simulink model "project_simu"  (R2019a)
settings: Solver=VariableStepAuto  StartTime=0.0  StopTime=1  RelTol=1e-3
values from neighbouring files (symbols this model uses):
  banks = 1e6*banks_data    [project.m]
  f = Filters/mean(Filters)    [project.m]
  lines = lines_data    [project.m]
  loads = zeros(10,2)    [project.m]
  m = 2    [project.m]
libraries: powerlib x87, powerlib_meascontrol x1, sps_avr x1
(part 2 of 2)

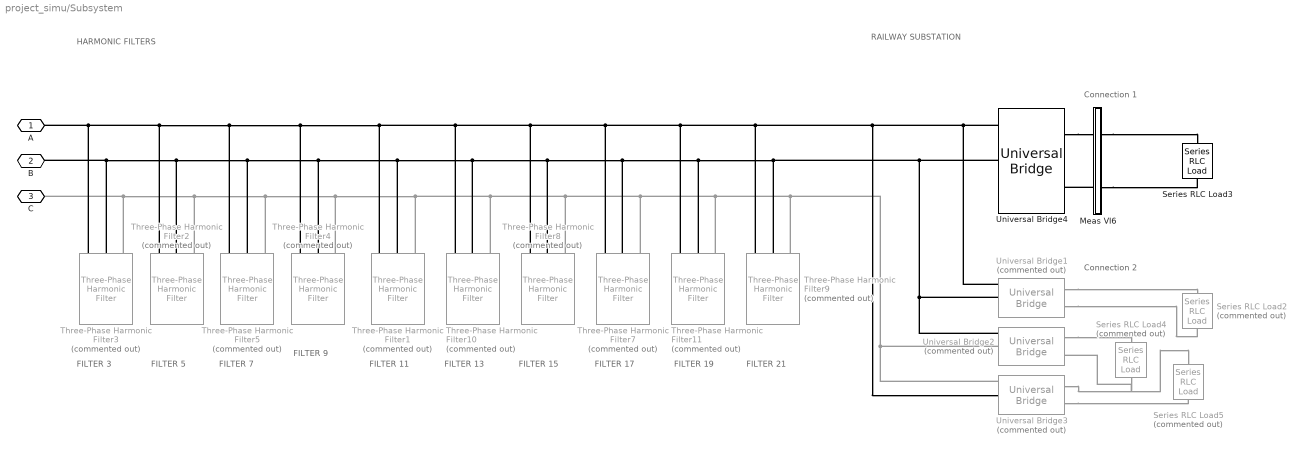
== system project_simu/Subsystem ==
  note: FILTER 5
  note: FILTER 11
  note: FILTER 3
  note: FILTER 9
  note: FILTER 7
  note: HARMONIC FILTERS
  note: RAILWAY SUBSTATION
  note: FILTER 17
  note: FILTER 15
  note: FILTER 21
  note: FILTER 13
  note: FILTER 19
  note: Connection 1
  note: Connection 2
  Meas VI6 : Subsystem
  Series RLC Load2 : powerlib/Elements/Series RLC Load  Commented=on  LConnTagsString=a  RConnTagsString=__new0  NominalVoltage=70e3*sqrt(2)  NominalFrequency=50  ActivePower=loads(10,1)/3  InductivePower=loads(10,2)/3  CapacitivePower=0  Setx0=off  InitialVoltage=0  SetiL0=off  InitialCurrent=0  Measurements=None  LoadType=constant Z
      settings: SourceProductName=Simscape Electrical
  Series RLC Load3 : powerlib/Elements/Series RLC Load  LConnTagsString=a  RConnTagsString=__new0  NominalVoltage=70e3*sqrt(2)  NominalFrequency=50  ActivePower=loads(10,1)  InductivePower=loads(10,2)  CapacitivePower=0  Setx0=off  InitialVoltage=0  SetiL0=off  InitialCurrent=0  Measurements=None  LoadType=constant Z
      settings: SourceProductName=Simscape Electrical
  Series RLC Load4 : powerlib/Elements/Series RLC Load  Commented=on  LConnTagsString=a  RConnTagsString=__new0  NominalVoltage=70e3*sqrt(2)  NominalFrequency=50  ActivePower=loads(10,1)/3  InductivePower=loads(10,2)/3  CapacitivePower=0  Setx0=off  InitialVoltage=0  SetiL0=off  InitialCurrent=0  Measurements=None  LoadType=constant Z
      settings: SourceProductName=Simscape Electrical
  Series RLC Load5 : powerlib/Elements/Series RLC Load  Commented=on  LConnTagsString=a  RConnTagsString=__new0  NominalVoltage=70e3*sqrt(2)  NominalFrequency=50  ActivePower=loads(10,1)/3  InductivePower=loads(10,2)/3  CapacitivePower=0  Setx0=off  InitialVoltage=0  SetiL0=off  InitialCurrent=0  Measurements=None  LoadType=constant Z
      settings: SourceProductName=Simscape Electrical
  Three-Phase Harmonic Filter1 : powerlib/Elements/Three-Phase Harmonic Filter  Commented=on  LConnTagsString=A|B|C  FilterType=Single-tuned  FilterConnection=Y (grounded)  ParNom=[70e3 50]  Qc=9e6*f(5)  Fr=[11*50]  Frd=[11*60 13*60]  Q=10  Measurements=None
      settings: AttributesFormatString=\n  SourceProductName=Simscape Electrical  SourceProductBaseCode=PS
  Three-Phase Harmonic Filter10 : powerlib/Elements/Three-Phase Harmonic Filter  Commented=on  LConnTagsString=A|B|C  FilterType=Single-tuned  FilterConnection=Y (grounded)  ParNom=[70e3 50]  Qc=9e6*f(6)  Fr=[13*50]  Frd=[11*60 13*60]  Q=10  Measurements=None
      settings: AttributesFormatString=\n  SourceProductName=Simscape Electrical  SourceProductBaseCode=PS
  Three-Phase Harmonic Filter11 : powerlib/Elements/Three-Phase Harmonic Filter  Commented=on  LConnTagsString=A|B|C  FilterType=Single-tuned  FilterConnection=Y (grounded)  ParNom=[70e3 50]  Qc=9e6*f(9)  Fr=[19*50]  Frd=[11*60 13*60]  Q=10  Measurements=None
      settings: AttributesFormatString=\n  SourceProductName=Simscape Electrical  SourceProductBaseCode=PS
  Three-Phase Harmonic Filter2 : powerlib/Elements/Three-Phase Harmonic Filter  Commented=on  LConnTagsString=A|B|C  FilterType=Single-tuned  FilterConnection=Y (grounded)  ParNom=[70e3 50]  Qc=9e6*f(2)  Fr=[5*50]  Frd=[266 323]  Q=10  Measurements=None
      settings: AttributesFormatString=\n  SourceProductName=Simscape Electrical  SourceProductBaseCode=PS
  Three-Phase Harmonic Filter3 : powerlib/Elements/Three-Phase Harmonic Filter  Commented=on  LConnTagsString=A|B|C  FilterType=Single-tuned  FilterConnection=Y (grounded)  ParNom=[70e3 50]  Qc=9e6*f(1)  Fr=[3*50]  Frd=[11*60 13*60]  Q=10  Measurements=None
      settings: AttributesFormatString=\n  SourceProductName=Simscape Electrical  SourceProductBaseCode=PS
  Three-Phase Harmonic Filter4 : powerlib/Elements/Three-Phase Harmonic Filter  Commented=on  LConnTagsString=A|B|C  FilterType=Single-tuned  FilterConnection=Y (grounded)  ParNom=[70e3 50]  Qc=9e6/9*f(4)  Fr=[9*50]  Frd=[11*60 13*60]  Q=10  Measurements=None
      settings: AttributesFormatString=\n  SourceProductName=Simscape Electrical  SourceProductBaseCode=PS
  Three-Phase Harmonic Filter5 : powerlib/Elements/Three-Phase Harmonic Filter  Commented=on  LConnTagsString=A|B|C  FilterType=Single-tuned  FilterConnection=Y (grounded)  ParNom=[70e3 50]  Qc=9e6/9*f(3)  Fr=[7*50]  Frd=[5*50 7*50]  Q=10  Measurements=None
      settings: AttributesFormatString=\n  SourceProductName=Simscape Electrical  SourceProductBaseCode=PS
  Three-Phase Harmonic Filter7 : powerlib/Elements/Three-Phase Harmonic Filter  Commented=on  LConnTagsString=A|B|C  FilterType=Single-tuned  FilterConnection=Y (grounded)  ParNom=[70e3 50]  Qc=9e6*f(8)  Fr=[17*50]  Frd=[11*60 13*60]  Q=10  Measurements=None
      settings: AttributesFormatString=\n  SourceProductName=Simscape Electrical  SourceProductBaseCode=PS
  Three-Phase Harmonic Filter8 : powerlib/Elements/Three-Phase Harmonic Filter  Commented=on  LConnTagsString=A|B|C  FilterType=Single-tuned  FilterConnection=Y (grounded)  ParNom=[70e3 50]  Qc=9e6*f(7)  Fr=[15*50]  Frd=[11*60 13*60]  Q=10  Measurements=None
      settings: AttributesFormatString=\n  SourceProductName=Simscape Electrical  SourceProductBaseCode=PS
  Three-Phase Harmonic Filter9 : powerlib/Elements/Three-Phase Harmonic Filter  Commented=on  LConnTagsString=A|B|C  FilterType=Single-tuned  FilterConnection=Y (grounded)  ParNom=[70e3 50]  Qc=9e6*f(10)  Fr=[21*50]  Frd=[11*60 13*60]  Q=10  Measurements=None
      settings: AttributesFormatString=\n  SourceProductName=Simscape Electrical  SourceProductBaseCode=PS
  Universal Bridge1 : powerlib/Power Electronics/Universal Bridge  Commented=on  Arms=3  SnubberResistance=1e5  SnubberCapacitance=inf  Device=Diodes  Ron=1e-3  Lon=0  ForwardVoltages="[  0  0  ]"  ForwardVoltage=0  GTOparameters=[ 10e-6 , 20e-6 ]  IGBTparameters=[ 1e-6 , 2e-6 ]  Measurements=None  Measurements_2=None  converterType=Rectifier
      settings: SourceProductName=Simscape Electrical
  Universal Bridge2 : powerlib/Power Electronics/Universal Bridge  Commented=on  Arms=3  SnubberResistance=1e5  SnubberCapacitance=inf  Device=Diodes  Ron=1e-3  Lon=0  ForwardVoltages="[  0  0  ]"  ForwardVoltage=0  GTOparameters=[ 10e-6 , 20e-6 ]  IGBTparameters=[ 1e-6 , 2e-6 ]  Measurements=None  Measurements_2=None  converterType=Rectifier
      settings: SourceProductName=Simscape Electrical
  Universal Bridge3 : powerlib/Power Electronics/Universal Bridge  Commented=on  Arms=3  SnubberResistance=1e5  SnubberCapacitance=inf  Device=Diodes  Ron=1e-3  Lon=0  ForwardVoltages="[  0  0  ]"  ForwardVoltage=0  GTOparameters=[ 10e-6 , 20e-6 ]  IGBTparameters=[ 1e-6 , 2e-6 ]  Measurements=None  Measurements_2=None  converterType=Rectifier
      settings: SourceProductName=Simscape Electrical
  Universal Bridge4 : powerlib/Power Electronics/Universal Bridge  Arms=3  SnubberResistance=1e5  SnubberCapacitance=inf  Device=Diodes  Ron=1e-3  Lon=0  ForwardVoltages="[  0  0  ]"  ForwardVoltage=0  GTOparameters=[ 10e-6 , 20e-6 ]  IGBTparameters=[ 1e-6 , 2e-6 ]  Measurements=None  Measurements_2=None  converterType=Rectifier
      settings: SourceProductName=Simscape Electrical
  A : PMIOPort  Side=Left
  B : PMIOPort  Port=2  Side=Left
  C : PMIOPort  Port=3  Side=Left
  connections:
  Three-Phase Harmonic Filter3/LConn3 -- C/RConn1 -- Universal Bridge3/LConn1 -- Universal Bridge2/LConn2 -- Three-Phase Harmonic Filter9/LConn3 -- Three-Phase Harmonic Filter11/LConn3 -- Three-Phase Harmonic Filter7/LConn3 -- Three-Phase Harmonic Filter8/LConn3 -- Three-Phase Harmonic Filter10/LConn3 -- Three-Phase Harmonic Filter1/LConn3 -- Three-Phase Harmonic Filter4/LConn3 -- Three-Phase Harmonic Filter5/LConn3 -- Three-Phase Harmonic Filter2/LConn3
  Three-Phase Harmonic Filter3/LConn2 -- B/RConn1 -- Three-Phase Harmonic Filter11/LConn2 -- Universal Bridge1/LConn2 -- Universal Bridge2/LConn1 -- Universal Bridge4/LConn2 -- Three-Phase Harmonic Filter9/LConn2 -- Three-Phase Harmonic Filter7/LConn2 -- Three-Phase Harmonic Filter8/LConn2 -- Three-Phase Harmonic Filter10/LConn2 -- Three-Phase Harmonic Filter1/LConn2 -- Three-Phase Harmonic Filter4/LConn2 -- Three-Phase Harmonic Filter5/LConn2 -- Three-Phase Harmonic Filter2/LConn2
  Three-Phase Harmonic Filter10/LConn1 -- Three-Phase Harmonic Filter11/LConn1 -- Universal Bridge1/LConn1 -- Universal Bridge4/LConn1 -- Universal Bridge3/LConn2 -- Three-Phase Harmonic Filter9/LConn1 -- Three-Phase Harmonic Filter7/LConn1 -- Three-Phase Harmonic Filter8/LConn1 -- Three-Phase Harmonic Filter1/LConn1 -- Three-Phase Harmonic Filter4/LConn1 -- Three-Phase Harmonic Filter5/LConn1 -- Three-Phase Harmonic Filter2/LConn1 -- Three-Phase Harmonic Filter3/LConn1 -- A/RConn1
  Universal Bridge1/RConn1 -- Series RLC Load2/LConn1
  Universal Bridge4/RConn1 -- Meas VI6/LConn1
  Meas VI6/RConn2 -- Series RLC Load3/RConn1
  Universal Bridge1/RConn2 -- Series RLC Load2/RConn1
  Universal Bridge2/RConn1 -- Series RLC Load4/LConn1
  Series RLC Load4/RConn1 -- Universal Bridge2/RConn2
  Universal Bridge3/RConn1 -- Series RLC Load5/LConn1
  Universal Bridge3/RConn2 -- Series RLC Load5/RConn1
  Meas VI6/RConn1 -- Series RLC Load3/LConn1
  Meas VI6/LConn2 -- Universal Bridge4/RConn2

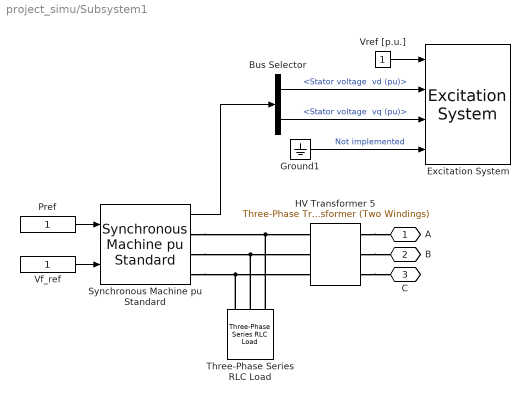
== system project_simu/Subsystem1 ==
  Bus Selector : BusSelector  OutputSignals="dq0 components.Stator voltage  vd (pu),dq0 components.Stator voltage  vq (pu)"
  Excitation System : sps_avr/Excitation System  tr=20e-3  reg=[ 70, 0.001 ]  exc=[ 1, 0 ]  tgr=[ 0, 0 ]  damp=[ 0.001, 0.1 ]  sat=[ 0, 0 ]  lim=[ -11.5, 11.5, 0 ]  v0="[1.0  1.28]"
      settings: SourceProductName=Simscape Electrical  SourceProductBaseCode=PS
  Ground1 : Ground
  HV Transformer 5 : powerlib/Elements/Three-Phase Transformer (Two Windings)  Winding1Connection=Yg  Winding2Connection=Yg  CoreType=Three single-phase transformers  SetSaturation=off  Hysteresis=off  DataFile='hysteresis'  SetInitialFlux=off  Measurements=None  UNITS=pu  NominalPower=[ 25e6 , 50 ]  Winding1=[6.5e3 0 0.05]  Winding2=[73e3 0 0.05]  Rm=500  Lm=500  L0=0.5  Saturation=[0 0;0.0024 1.2;0.99998 1.52]  InitialFluxes=[ 0.8 , -0.8 , 0.7 ]  BreakLoop=off  DiscreteSolver=Trapezoidal iterative  DataType=off  TransfoNumber=1
      settings: SourceProductName=Simscape Electrical
  Pref : Constant
  Synchronous Machine pu Standard : powerlib/Machines/Synchronous Machine pu Standard  PresetModel=No  MechanicalLoad=Mechanical power Pm  ShowDetailedParameters=on  RotorType=Round  Units=per unit standard parameters  MeasurementBus=off  NominalParameters=[25e6 6e3 50]  Reactances1=[ 1.81, 0.3, 0.23, 1.76, 0.65, 0.25, 0.15 ]  Reactances2=[1.83 0.30 0.23 1.02 0.13 0.08]  dAxisTimeConstants=Short-circuit  qAxisTimeConstants=Short-circuit  TimeConstants1="[ 4.4849  0.0681  0.1  ]"  TimeConstants2=[ 8.0, 0.03, 1.0, 0.07 ]  TimeConstants3="[  4.49  0.0681  0.0513  ]"  TimeConstants4=[ 8.0, 0.03, 0.3371, 0.0295 ]  TimeConstants5=[ 1.01, 0.053, 0.1 ]  TimeConstants6=[ 1.3201, 0.023, 1.0, 0.07 ]  TimeConstants7=[0.012 0.003 0.003]  TimeConstants8=[ 1.3201, 0.0231, 0.3371, 0.0295 ]  StatorResistance=0.037875  Mechanical=[0.1028 0.02056 2]  PolePairs=20  InitialConditions="[ 0 -70  0 0 0  0  -120  120  1 ]"  SetSaturation=off  Saturation=[0.6404,0.7127,0.8441,0.9214,0.9956,1.082,1.19,1.316,1.457;0.7,0.7698,0.8872,0.9466,0.9969,1.046,1.1,1.151,1.201]  LoadFlowParameters=[1,0,0,0,0]  TsPowergui=0  TsBlock=-1  IterativeModel=Trapezoidal non iterative  IterativeDiscreteModel=Trapezoidal non iterative  BusType=PQ  Pref=0  Qref=0  Qmin=-inf  Qmax=inf  PLF=0  QLF=0
      settings: SourceProductName=Simscape Electrical
  Three-Phase Series RLC Load : powerlib/Elements/Three-Phase Series RLC Load  LConnTagsString=A|B|C  Configuration=Y (grounded)  NominalVoltage=6e3  Vabc=[1e3 1e3 1e3]  Vabcp=[1e3 1e3 1e3]  NominalFrequency=50  UnbalancedPower=off  ActivePower=1  InductivePower=0  CapacitivePower=0  Pabc=[10e3 9e3 11e3]  QLabc=[100 90 110]  QCabc=[100 90 110]  Pabcp=[10e3 9e3 11e3]  QLabcp=[100 90 110]  QCabcp=[100 90 110]  Measurements=None  LoadType=constant Z
      settings: SourceProductName=Simscape Electrical
  Vf_ref : Constant
  Vref [p.u.] : Constant
  A : PMIOPort  Side=Right
  B : PMIOPort  Port=2  Side=Right
  C : PMIOPort  Port=3  Side=Right
  wires:
  Pref/1 -> Synchronous Machine pu Standard/1
  Synchronous Machine pu Standard/1 -> Bus Selector/1
  Vref [p.u.]/1 -> Excitation System/1
  Bus Selector/1 -> Excitation System/2  "<Stator voltage  vd (pu)>"
  Bus Selector/2 -> Excitation System/3  "<Stator voltage  vq (pu)>"
  Ground1/1 -> Excitation System/4  "Not implemented"
  Vf_ref/1 -> Synchronous Machine pu Standard/2
  connections:
  Synchronous Machine pu Standard/RConn1 -- Three-Phase Series RLC Load/LConn1 -- HV Transformer 5/LConn1
  HV Transformer 5/RConn1 -- A/RConn1
  Synchronous Machine pu Standard/RConn3 -- Three-Phase Series RLC Load/LConn3 -- HV Transformer 5/LConn3
  HV Transformer 5/RConn3 -- C/RConn1
  Synchronous Machine pu Standard/RConn2 -- HV Transformer 5/LConn2 -- Three-Phase Series RLC Load/LConn2
  HV Transformer 5/RConn2 -- B/RConn1

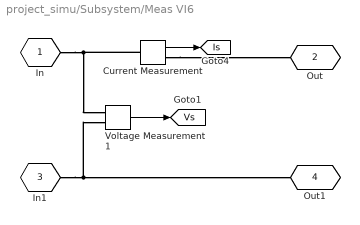
== system project_simu/Subsystem/Meas VI6 ==
  Current Measurement : powerlib/Measurements/Current Measurement  PhasorSimulation=off  OutputType=Complex  PSBequivalent=0
      settings: SourceProductName=Simscape Electrical
  Voltage Measurement1 : powerlib/Measurements/Voltage Measurement  Tag=PoWeRsYsTeMmEaSuReMeNt  PhasorSimulation=off  OutputType=Magnitude  PSBequivalent=0
      settings: SourceProductName=Simscape Electrical
  In : PMIOPort  Tag=PMCPort  Side=Left
  Out : PMIOPort  Tag=PMCPort  Port=2  Side=Right
  In1 : PMIOPort  Tag=PMCPort  Port=3  Side=Left
  Out1 : PMIOPort  Tag=PMCPort  Port=4  Side=Right
  tag scope: Is=global, Vs=global
  wires:
  Voltage Measurement1/1 -> [Vs]
  Current Measurement/1 -> [Is]
  connections:
  Current Measurement/RConn1 -- Out/RConn1
  Current Measurement/LConn1 -- Voltage Measurement1/LConn1 -- In/RConn1
  In1/RConn1 -- Out1/RConn1 -- Voltage Measurement1/LConn2
